simulink model "psbigbtconv"  (Simulink 6.0)
settings: Solver=ode23tb  StartTime=0.0  StopTime=20e-3  RelTol=1e-3  AbsTol=1e-3
InitFcn:
  | powericon('psbinitsys',bdroot);
libraries: powerlib2 x8, simulink x1
settings Model: Creator=batserve  LastModifiedBy=batserve  ExtModeTrigMode=oneshot  ExtModeArmWhenConnect=off  ExtModeAutoUpdateStatusClock=off
settings DataIOCC: LimitDataPoints=off
settings OptimizationCC: BlockReduction=off  BooleanDataType=off
settings DebuggingCC: SolverPrmCheckMsg=none
settings HardwareCC: TargetUnknown=on

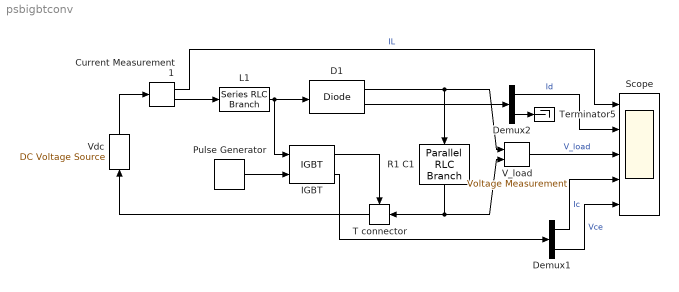
== system psbigbtconv ==
  Current Measurement1 : powerlib2/Measurements/Current Measurement  Tag=PoWeRsYsTeMmEaSuReMeNt  PSBOutputType=01  PSBequivalent=0
  D1 : powerlib2/Power Electronics/Diode  Tag=PoWeRsYsTeMbLoCk  Ron=0.05  Lon=0.1e-6  Vf=0.8  IC=0  Rs=1e5  Cs=inf  PSBOutputType=10
  Demux1 : Demux  Outputs=2
  Demux2 : Demux  Outputs=2
  IGBT : powerlib2/Power Electronics/IGBT  Tag=PoWeRsYsTeMbLoCk  Ron=0.01  Lon=1e-6  Vf=1  Tf=1e-6  Tt=1e-6  IC=0  Rs=10000  Cs=inf  PSBOutputType=10
  L1 : powerlib2/Elements/Series RLC Branch  Tag=PoWeRsYsTeMbLoCk  a=0  b=400e-6  c=inf  mesure=None  PSBOutputType=1
  Pulse Generator : simulink/Sources/Pulse Generator  period=100e-6  duty=50  amplitude=1  start=0
  R1 C1 : powerlib2/Elements/Parallel RLC Branch  Tag=PoWeRsYsTeMbLoCk  Orientation=down  a=50  b=inf  c=25e-06  mesure=None  PSBOutputType=1
  Scope : Scope  NumInputPorts=5
      settings: TimeRange=0.02  YMin=-10~0~0~0~0  YMax=70~70~400~70~700  SaveName=var  MaxDataPoints=50000
  T connector : powerlib2/Connectors/T connector  Tag=PoWeRsYsTeMbLoCk  Orientation=left  PSBOutputType=1
  Terminator5 : Terminator
  V_load : powerlib2/Measurements/Voltage Measurement  Tag=PoWeRsYsTeMmEaSuReMeNt  PSBOutputType=0  PSBequivalent=0
  Vdc : powerlib2/Electrical Sources/DC Voltage Source  Tag=PoWeRsYsTeMbLoCk  Description=source block  Orientation=up  V=100  mesure=None  PSBOutputType=1
  wires:
  D1/1 -> R1 C1/1, V_load/1
  IGBT/2 -> Demux1/1
  R1 C1/1 -> V_load/2, T connector/1
  T connector/1 -> Vdc/1
  IGBT/1 -> T connector/Enable
  Pulse Generator/1 -> IGBT/2
  Current Measurement1/2 -> L1/1
  Vdc/1 -> Current Measurement1/1
  L1/1 -> IGBT/1, D1/1
  Current Measurement1/1 -> Scope/1  "IL"
  D1/2 -> Demux2/1
  Demux2/2 -> Terminator5/1
  Demux2/1 -> Scope/2  "Id"
  V_load/1 -> Scope/3  "V_load"
  Demux1/1 -> Scope/4  "Ic"
  Demux1/2 -> Scope/5  "Vce"
